simulink model "GlucagonInsulinIntegration"  (R2019a)
settings: Solver=VariableStepAuto  StartTime=0.0  StopTime=10  RelTol=1e-3
undefined symbols (not defined in the file): ILC_B, IPT_B
settings Model: Creator=rache  LastModifiedBy=rache

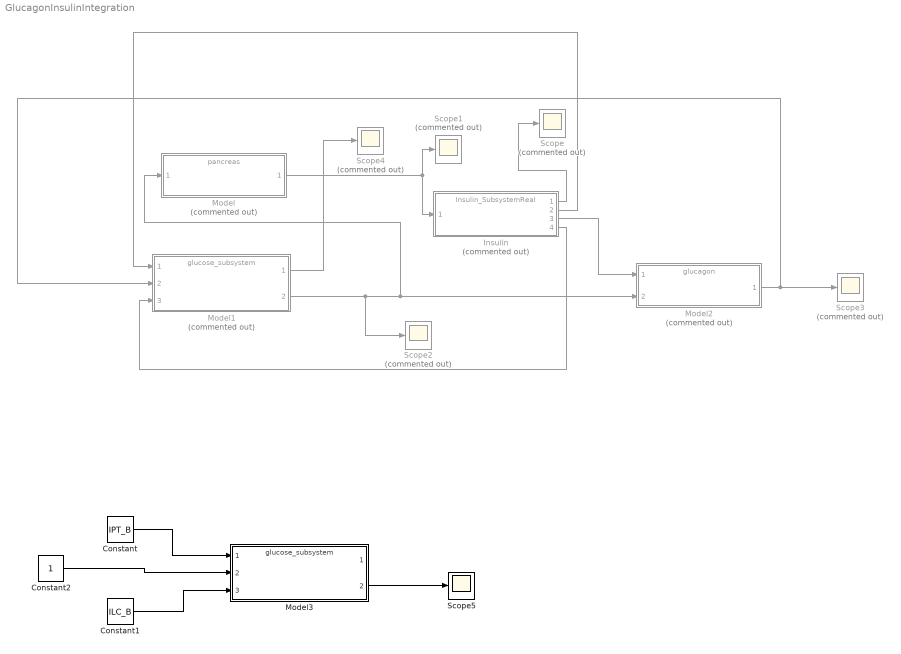
== system GlucagonInsulinIntegration ==
  Constant : Constant  Value=IPT_B
  Constant1 : Constant  Value=ILC_B
  Constant2 : Constant
  Insulin : ModelReference  Commented=on  ModelNameDialog=Insulin_SubsystemReal  SimulationMode=Normal  ModelReferenceVersion=1.40
  Model : ModelReference  Commented=on  ModelNameDialog=pancreas  SimulationMode=Normal  ModelReferenceVersion=1.16
  Model1 : ModelReference  Commented=on  ModelNameDialog=glucose_subsystem  SimulationMode=Normal  ModelReferenceVersion=1.45
  Model2 : ModelReference  Commented=on  ModelNameDialog=glucagon  SimulationMode=Normal  ModelReferenceVersion=1.9
  Model3 : ModelReference  ModelNameDialog=glucose_subsystem  SimulationMode=Normal  ModelReferenceVersion=1.45
  Scope{,1..4} (5 alike) : Scope  Commented=on
  Scope5 : Scope
  wires:
  Model/1 -> Insulin/1, Scope1/1
  Insulin/1 -> Scope/1
  Model1/2 -> Scope2/1, Model/1, Model2/2
  Insulin/3 -> Model2/1
  Model2/1 -> Scope3/1, Model1/2
  Insulin/2 -> Model1/1
  Insulin/4 -> Model1/3
  Model1/1 -> Scope4/1
  Model3/2 -> Scope5/1
  Constant1/1 -> Model3/3
  Constant/1 -> Model3/1
  Constant2/1 -> Model3/2
